simulink model "ControlsWithAutopilot_NoBus_PP_Discrete_Fcn_Atomic"  (Simulink 7.2)
settings: Solver=ode45  StartTime=0.0  StopTime=10.0  RelTol=1e-3
undefined symbols (not defined in the file): ap, bias, DiscIntNeverNeededParam
libraries: simulink x3, discretizing x1
(part 2 of 2)

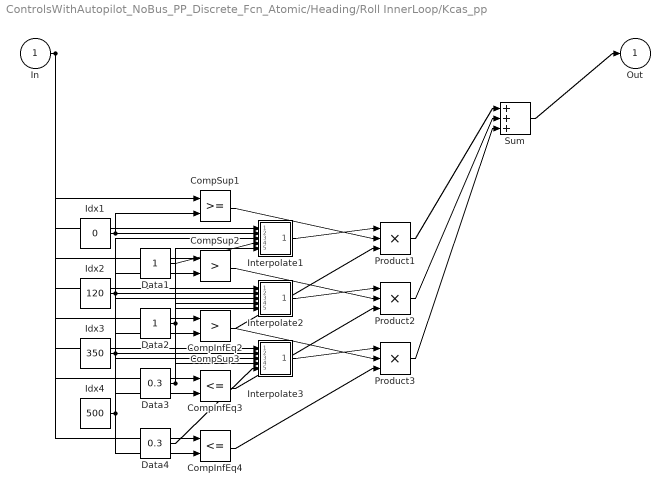
== system ControlsWithAutopilot_NoBus_PP_Discrete_Fcn_Atomic/Heading/Roll InnerLoop/Kcas_pp ==
  In : Inport
  CompInfEq2 : RelationalOperator  Operator=<=  InputSameDT=on
  CompInfEq3 : RelationalOperator  Operator=<=  InputSameDT=on
  CompInfEq4 : RelationalOperator  Operator=<=  InputSameDT=on
  CompSup1 : RelationalOperator  InputSameDT=on
  CompSup2 : RelationalOperator  Operator=>  InputSameDT=on
  CompSup3 : RelationalOperator  Operator=>  InputSameDT=on
  Data1 : Constant
  Data2 : Constant
  Data3 : Constant  Value=0.3
  Data4 : Constant  Value=0.3
  Idx1 : Constant  Value=0
  Idx2 : Constant  Value=120
  Idx3 : Constant  Value=350
  Idx4 : Constant  Value=500
  Interpolate1 : Subsystem
  Interpolate2 : Subsystem
  Interpolate3 : Subsystem
  Product1 : Product  Inputs=***  SaturateOnIntegerOverflow=on  RndMeth=Zero  OutDataTypeStr=Inherit: Same as first input
  Product2 : Product  Inputs=***  SaturateOnIntegerOverflow=on  RndMeth=Zero  OutDataTypeStr=Inherit: Same as first input
  Product3 : Product  Inputs=***  SaturateOnIntegerOverflow=on  RndMeth=Zero  OutDataTypeStr=Inherit: Same as first input
  Sum : Sum  Inputs=+++  SaturateOnIntegerOverflow=on  InputSameDT=on  OutDataTypeStr=Inherit: Same as first input
  Out : Outport
  wires:
  In/1 -> Interpolate1/1(InportIn), CompSup1/1, Interpolate2/1(InportIn), CompSup2/1, CompInfEq2/1, Interpolate3/1(InportIn), CompSup3/1, CompInfEq3/1, CompInfEq4/1
  Idx1/1 -> Interpolate1/2(InportIdx1), CompSup1/2
  Data1/1 -> Interpolate1/4(InportData1)
  Interpolate1/1(Out) -> Product1/1
  CompSup1/1 -> Product1/2
  CompInfEq2/1 -> Product1/3
  Product1/1 -> Sum/1
  Idx2/1 -> Interpolate2/2(InportIdx1), CompSup2/2, Interpolate1/3(InportIdx2), CompInfEq2/2
  Data2/1 -> Interpolate2/4(InportData1), Interpolate1/5(InportData2)
  Interpolate2/1(Out) -> Product2/1
  CompSup2/1 -> Product2/2
  CompInfEq3/1 -> Product2/3
  Product2/1 -> Sum/2
  Idx3/1 -> Interpolate3/2(InportIdx1), CompSup3/2, Interpolate2/3(InportIdx2), CompInfEq3/2
  Data3/1 -> Interpolate3/4(InportData1), Interpolate2/5(InportData2)
  Interpolate3/1(Out) -> Product3/1
  CompSup3/1 -> Product3/2
  CompInfEq4/1 -> Product3/3
  Product3/1 -> Sum/3
  Idx4/1 -> Interpolate3/3(InportIdx2), CompInfEq4/2
  Data4/1 -> Interpolate3/5(InportData2)
  Sum/1 -> Out/1

== system ControlsWithAutopilot_NoBus_PP_Discrete_Fcn_Atomic/Longitudinal/Altitude Control/Variable  Rate Limit ==
  ratelim : Inport  RequirementInfo={} %GIDa_1ef85aab_f902_404e_a68b_00e57673dd3f
  input : Inport  RequirementInfo={} %GIDa_7ac59940_1fcc_4039_a5aa_a007950c590e  Port=2
  ICtrig : Inport  RequirementInfo={} %GIDa_9850dee7_08ca_49d5_88fb_399ee4ba203e  Port=3
  IC : Inport  RequirementInfo={} %GIDa_d80fe626_91fd_4f82_ad17_86aca6b3aee5  Port=4
  Gain : Gain  RequirementInfo={} %GIDa_55467e41_3bd6_44bf_9a44_6f78661bf8f0  Gain=20  SaturateOnIntegerOverflow=on  OutDataTypeStr=Inherit: Same as input  ParamDataTypeStr=Inherit: Same as input
  Gain1 : Gain  RequirementInfo={} %GIDa_0b7dd2e9_dfcf_42d3_8fb1_8c254e005ceb  Gain=-1  SaturateOnIntegerOverflow=on  OutDataTypeStr=Inherit: Same as input  ParamDataTypeStr=Inherit: Same as input
  Integrator : DiscreteIntegrator  ExternalReset=level  InitialConditionSource=external  SampleTime=1.0  ICPrevOutput=DiscIntNeverNeededParam  ICPrevScaledInput=DiscIntNeverNeededParam  mask(DiscretizedDiscreteIntegrator){}
      mask init:
      | %zoh
  Sum2 : Sum  RequirementInfo={} %GIDa_de9ff84b_54f5_48bc_9ef3_874415208380  Inputs=|+-  SaturateOnIntegerOverflow=on
  Variable Limit Saturation : Subsystem  RequirementInfo={} %GIDa_42540829_63e9_4d83_adf5_d7c684208c2d
  output : Outport  RequirementInfo={} %GIDa_74eb2916_410f_4b2d_afdf_0d476e7e03b7
  wires:
  Sum2/1 -> Gain/1
  Gain/1 -> Variable Limit Saturation/2(SigIn)
  ratelim/1 -> Gain1/1, Variable Limit Saturation/1(up_lim)
  Gain1/1 -> Variable Limit Saturation/3(Lo_lim)
  Variable Limit Saturation/1(Out1) -> Integrator/1
  Integrator/1 -> Sum2/2, output/1
  input/1 -> Sum2/1
  ICtrig/1 -> Integrator/2
  IC/1 -> Integrator/3

== system ControlsWithAutopilot_NoBus_PP_Discrete_Fcn_Atomic/Longitudinal/Altitude Control/Variable Limit Saturation ==
  up_lim : Inport  RequirementInfo={} %GIDa_a8c5a358_1294_4ae6_a63f_3940fe218386
  SigIn : Inport  RequirementInfo={} %GIDa_062a0af8_40f0_4204_856b_8e0aded8de05  Port=2
  Lo_lim : Inport  RequirementInfo={} %GIDa_6793747b_c094_4bd9_a5cb_839f8eb54e21  Port=3
  Enforce low lim : MinMax  RequirementInfo={} %GIDa_e93f4b97_2f8b_4f52_84c9_3cb68ddf7e16  Function=max  Inputs=2
  Enforce up lim : MinMax  RequirementInfo={} %GIDa_c018e6ad_c664_4361_a96c_d990e2efb7d8  Inputs=2
  Out1 : Outport  RequirementInfo={} %GIDa_0d7a9d35_dde5_41a4_a708_f2de214bfa54
  wires:
  Lo_lim/1 -> Enforce low lim/1
  SigIn/1 -> Enforce low lim/2
  Enforce low lim/1 -> Enforce up lim/1
  up_lim/1 -> Enforce up lim/2
  Enforce up lim/1 -> Out1/1

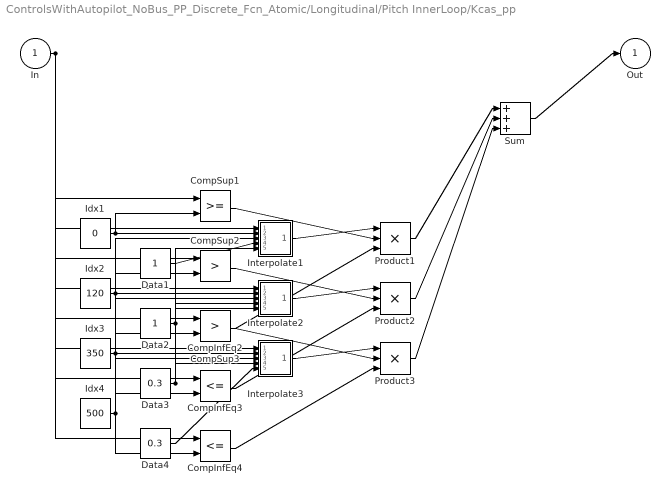
== system ControlsWithAutopilot_NoBus_PP_Discrete_Fcn_Atomic/Longitudinal/Pitch InnerLoop/Kcas_pp ==
  In : Inport
  CompInfEq2 : RelationalOperator  Operator=<=  InputSameDT=on
  CompInfEq3 : RelationalOperator  Operator=<=  InputSameDT=on
  CompInfEq4 : RelationalOperator  Operator=<=  InputSameDT=on
  CompSup1 : RelationalOperator  InputSameDT=on
  CompSup2 : RelationalOperator  Operator=>  InputSameDT=on
  CompSup3 : RelationalOperator  Operator=>  InputSameDT=on
  Data1 : Constant
  Data2 : Constant
  Data3 : Constant  Value=0.3
  Data4 : Constant  Value=0.3
  Idx1 : Constant  Value=0
  Idx2 : Constant  Value=120
  Idx3 : Constant  Value=350
  Idx4 : Constant  Value=500
  Interpolate1 : Subsystem
  Interpolate2 : Subsystem
  Interpolate3 : Subsystem
  Product1 : Product  Inputs=***  SaturateOnIntegerOverflow=on  RndMeth=Zero  OutDataTypeStr=Inherit: Same as first input
  Product2 : Product  Inputs=***  SaturateOnIntegerOverflow=on  RndMeth=Zero  OutDataTypeStr=Inherit: Same as first input
  Product3 : Product  Inputs=***  SaturateOnIntegerOverflow=on  RndMeth=Zero  OutDataTypeStr=Inherit: Same as first input
  Sum : Sum  Inputs=+++  SaturateOnIntegerOverflow=on  InputSameDT=on  OutDataTypeStr=Inherit: Same as first input
  Out : Outport
  wires:
  In/1 -> Interpolate1/1(InportIn), CompSup1/1, Interpolate2/1(InportIn), CompSup2/1, CompInfEq2/1, Interpolate3/1(InportIn), CompSup3/1, CompInfEq3/1, CompInfEq4/1
  Idx1/1 -> Interpolate1/2(InportIdx1), CompSup1/2
  Data1/1 -> Interpolate1/4(InportData1)
  Interpolate1/1(Out) -> Product1/1
  CompSup1/1 -> Product1/2
  CompInfEq2/1 -> Product1/3
  Product1/1 -> Sum/1
  Idx2/1 -> Interpolate2/2(InportIdx1), CompSup2/2, Interpolate1/3(InportIdx2), CompInfEq2/2
  Data2/1 -> Interpolate2/4(InportData1), Interpolate1/5(InportData2)
  Interpolate2/1(Out) -> Product2/1
  CompSup2/1 -> Product2/2
  CompInfEq3/1 -> Product2/3
  Product2/1 -> Sum/2
  Idx3/1 -> Interpolate3/2(InportIdx1), CompSup3/2, Interpolate2/3(InportIdx2), CompInfEq3/2
  Data3/1 -> Interpolate3/4(InportData1), Interpolate2/5(InportData2)
  Interpolate3/1(Out) -> Product3/1
  CompSup3/1 -> Product3/2
  CompInfEq4/1 -> Product3/3
  Product3/1 -> Sum/3
  Idx4/1 -> Interpolate3/3(InportIdx2), CompInfEq4/2
  Data4/1 -> Interpolate3/5(InportData2)
  Sum/1 -> Out/1

== system ControlsWithAutopilot_NoBus_PP_Discrete_Fcn_Atomic/Longitudinal/Pitch InnerLoop/Transfer Fcn_pp ==
  Inport1 : Inport
  D1 : UnitDelay  SampleTime=-1
  GainAC1_1 : Gain  Gain=-0.0625  SaturateOnIntegerOverflow=on  OutDataTypeStr=Inherit: Same as input  ParamDataTypeStr=Inherit: Same as input
  GainAC2_1 : Gain  Gain=-0.0625  SaturateOnIntegerOverflow=on  OutDataTypeStr=Inherit: Same as input  ParamDataTypeStr=Inherit: Same as input
  GainBD1_1 : Gain  SaturateOnIntegerOverflow=on  OutDataTypeStr=Inherit: Same as input  ParamDataTypeStr=Inherit: Same as input
  GainBD2_1 : Gain  SaturateOnIntegerOverflow=on  OutDataTypeStr=Inherit: Same as input  ParamDataTypeStr=Inherit: Same as input
  Sum1 : Sum  SaturateOnIntegerOverflow=on  InputSameDT=on  OutDataTypeStr=Inherit: Same as first input
  Sum2 : Sum  SaturateOnIntegerOverflow=on  InputSameDT=on  OutDataTypeStr=Inherit: Same as first input
  Outport1 : Outport
  wires:
  D1/1 -> GainAC1_1/1, GainAC2_1/1
  GainAC1_1/1 -> Sum1/1
  GainAC2_1/1 -> Sum2/1
  Inport1/1 -> GainBD1_1/1, GainBD2_1/1
  GainBD1_1/1 -> Sum1/2
  GainBD2_1/1 -> Sum2/2
  Sum1/1 -> D1/1
  Sum2/1 -> Outport1/1

== system ControlsWithAutopilot_NoBus_PP_Discrete_Fcn_Atomic/Yaw Damper/Kcas_pp/Interpolate1 ==
  InportIn : Inport
  InportIdx1 : Inport  Port=2
  InportIdx2 : Inport  Port=3
  InportData1 : Inport  Port=4
  InportData2 : Inport  Port=5
  Interpolate : Product  Inputs=*/*  SaturateOnIntegerOverflow=on  RndMeth=Zero  InputSameDT=on  OutDataTypeStr=Inherit: Same as first input
  Sum1 : Sum  Inputs=+-  SaturateOnIntegerOverflow=on  InputSameDT=on  OutDataTypeStr=Inherit: Same as first input
  Sum2 : Sum  Inputs=-+  SaturateOnIntegerOverflow=on  InputSameDT=on  OutDataTypeStr=Inherit: Same as first input
  Sum3 : Sum  Inputs=-+  SaturateOnIntegerOverflow=on  InputSameDT=on  OutDataTypeStr=Inherit: Same as first input
  Sum4 : Sum  SaturateOnIntegerOverflow=on  InputSameDT=on  OutDataTypeStr=Inherit: Same as first input
  Out : Outport
  wires:
  InportIn/1 -> Sum1/1
  InportIdx1/1 -> Sum1/2, Sum2/1
  InportIdx2/1 -> Sum2/2
  InportData1/1 -> Sum3/1, Sum4/2
  InportData2/1 -> Sum3/2
  Sum1/1 -> Interpolate/1
  Sum2/1 -> Interpolate/2
  Sum3/1 -> Interpolate/3
  Interpolate/1 -> Sum4/1
  Sum4/1 -> Out/1

== system ControlsWithAutopilot_NoBus_PP_Discrete_Fcn_Atomic/Yaw Damper/Kcas_pp/Interpolate2 ==
  InportIn : Inport
  InportIdx1 : Inport  Port=2
  InportIdx2 : Inport  Port=3
  InportData1 : Inport  Port=4
  InportData2 : Inport  Port=5
  Interpolate : Product  Inputs=*/*  SaturateOnIntegerOverflow=on  RndMeth=Zero  InputSameDT=on  OutDataTypeStr=Inherit: Same as first input
  Sum1 : Sum  Inputs=+-  SaturateOnIntegerOverflow=on  InputSameDT=on  OutDataTypeStr=Inherit: Same as first input
  Sum2 : Sum  Inputs=-+  SaturateOnIntegerOverflow=on  InputSameDT=on  OutDataTypeStr=Inherit: Same as first input
  Sum3 : Sum  Inputs=-+  SaturateOnIntegerOverflow=on  InputSameDT=on  OutDataTypeStr=Inherit: Same as first input
  Sum4 : Sum  SaturateOnIntegerOverflow=on  InputSameDT=on  OutDataTypeStr=Inherit: Same as first input
  Out : Outport
  wires:
  InportIn/1 -> Sum1/1
  InportIdx1/1 -> Sum1/2, Sum2/1
  InportIdx2/1 -> Sum2/2
  InportData1/1 -> Sum3/1, Sum4/2
  InportData2/1 -> Sum3/2
  Sum1/1 -> Interpolate/1
  Sum2/1 -> Interpolate/2
  Sum3/1 -> Interpolate/3
  Interpolate/1 -> Sum4/1
  Sum4/1 -> Out/1

== system ControlsWithAutopilot_NoBus_PP_Discrete_Fcn_Atomic/Yaw Damper/Kcas_pp/Interpolate3 ==
  InportIn : Inport
  InportIdx1 : Inport  Port=2
  InportIdx2 : Inport  Port=3
  InportData1 : Inport  Port=4
  InportData2 : Inport  Port=5
  Interpolate : Product  Inputs=*/*  SaturateOnIntegerOverflow=on  RndMeth=Zero  InputSameDT=on  OutDataTypeStr=Inherit: Same as first input
  Sum1 : Sum  Inputs=+-  SaturateOnIntegerOverflow=on  InputSameDT=on  OutDataTypeStr=Inherit: Same as first input
  Sum2 : Sum  Inputs=-+  SaturateOnIntegerOverflow=on  InputSameDT=on  OutDataTypeStr=Inherit: Same as first input
  Sum3 : Sum  Inputs=-+  SaturateOnIntegerOverflow=on  InputSameDT=on  OutDataTypeStr=Inherit: Same as first input
  Sum4 : Sum  SaturateOnIntegerOverflow=on  InputSameDT=on  OutDataTypeStr=Inherit: Same as first input
  Out : Outport
  wires:
  InportIn/1 -> Sum1/1
  InportIdx1/1 -> Sum1/2, Sum2/1
  InportIdx2/1 -> Sum2/2
  InportData1/1 -> Sum3/1, Sum4/2
  InportData2/1 -> Sum3/2
  Sum1/1 -> Interpolate/1
  Sum2/1 -> Interpolate/2
  Sum3/1 -> Interpolate/3
  Interpolate/1 -> Sum4/1
  Sum4/1 -> Out/1

== system ControlsWithAutopilot_NoBus_PP_Discrete_Fcn_Atomic/Heading/Heading Control/HdgCmdProcessor/ANGL ==
  in : Inport  RequirementInfo={} %GIDa_91f853c7_c908_401d_adfc_518d7751528f
  Abs : Abs  OutDataType=sfix(16)  OutScaling=2^0
  Constant : Constant  Value=360  OutDataType=sfix(16)  OutScaling=2^0
  Constant1 : Constant  RequirementInfo={} %GIDa_7c5c3c02_b72b_4cab_88d9_ce8964dea6e5  Value=180
  Product : Product  OutDataType=sfix(16)  OutScaling=2^0  RndMeth=Zero
  Relational Operator : RelationalOperator  RequirementInfo={} %GIDa_7fca63f4_30c3_4611_a13c_f242258541ac  Operator=>
  Relational Operator1 : RelationalOperator  Operator=<  LogicOutDataTypeMode=boolean  OutDataTypeStr=boolean
  Sum6 : Sum  RequirementInfo={} %GIDa_8f691f86_6b2c_4343_a08d_01121fff99a8  Inputs=|-+  SaturateOnIntegerOverflow=on
  Switch1 : Switch  RequirementInfo={} %GIDa_9f6a3e17_ac1f_4a7c_b770_43e31d539b0d  Threshold=0.1  SaturateOnIntegerOverflow=on
  zero : Constant  Value=0  OutDataType=sfix(16)  OutScaling=2^0
  180 : Outport  RequirementInfo={} %GIDa_da671ccf_1469_4f90_9911_e50416dafc2f
  wires:
  Abs/1 -> Relational Operator/1
  in/1 -> Abs/1, Switch1/3, Sum6/2, Relational Operator1/2
  Switch1/1 -> 180/1
  Product/1 -> Sum6/1
  Sum6/1 -> Switch1/1
  Relational Operator/1 -> Switch1/2
  Constant1/1 -> Relational Operator/2
  zero/1 -> Relational Operator1/1
  Constant/1 -> Product/1
  Relational Operator1/1 -> Product/2

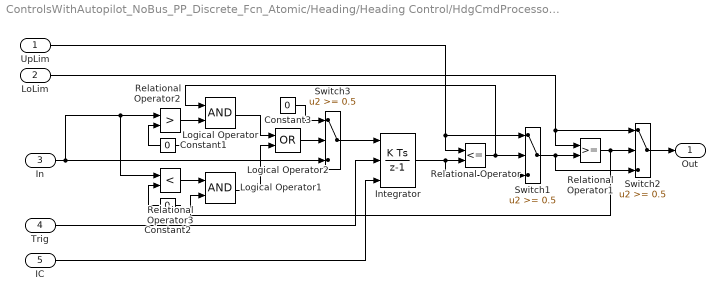
== system ControlsWithAutopilot_NoBus_PP_Discrete_Fcn_Atomic/Heading/Heading Control/HdgCmdProcessor/VarLimIntegIC ==
  UpLim : Inport  RequirementInfo={} %GIDa_b6974814_32b4_446c_a7b5_2b64616822d2
  LoLim : Inport  RequirementInfo={} %GIDa_b4069f0f_04d2_435d_9d74_47f31e226abc  Port=2
  In : Inport  RequirementInfo={} %GIDa_ffe63698_9663_4b08_a6c4_0cfcc14ab018  Port=3
  Trig : Inport  RequirementInfo={} %GIDa_6297cb9d_5b31_4d8e_a321_41fbf142c5b4  Port=4
  IC : Inport  RequirementInfo={} %GIDa_59f2d505_3cc2_4942_9dd8_a5a4ff923eba  Port=5
  Constant1 : Constant  RequirementInfo={} %GIDa_5f63bf18_9b52_4c75_b33f_d083ba316d1e  Value=0
  Constant2 : Constant  RequirementInfo={} %GIDa_3ef1a0c3_325a_4a1e_87f1_8a7ceb7f2ed7  Value=0
  Constant3 : Constant  RequirementInfo={} %GIDa_3c010cc6_e66d_42da_9a5a_231ebe5e9c3f  Value=0
  Integrator : DiscreteIntegrator  ExternalReset=level  InitialConditionSource=external  SampleTime=1.0  ICPrevOutput=DiscIntNeverNeededParam  ICPrevScaledInput=DiscIntNeverNeededParam  mask(DiscretizedDiscreteIntegrator){}
      mask init:
      | %zoh
  Logical Operator : Logic  RequirementInfo={} %GIDa_a60b4d2f_6552_4cb5_b522_727de66498b0  AllPortsSameDT=off
  Logical Operator1 : Logic  RequirementInfo={} %GIDa_8f81d6cf_a2aa_4e00_869d_ceffbd7871c1  AllPortsSameDT=off
  Logical Operator2 : Logic  RequirementInfo={} %GIDa_6338745d_e0be_46bf_a46f_644f808dad4e  Operator=OR  AllPortsSameDT=off
  Relational Operator : RelationalOperator  RequirementInfo={} %GIDa_8e878cd0_b3b2_4162_9fe2_c686049f0806  Operator=<=
  Relational Operator1 : RelationalOperator  RequirementInfo={} %GIDa_b45a0ded_1a8c_4a6d_a67f_e5d263373459
  Relational Operator2 : RelationalOperator  RequirementInfo={} %GIDa_a0755ed8_a69f_4262_8ce5_c41fc56502ff  Operator=>
  Relational Operator3 : RelationalOperator  RequirementInfo={} %GIDa_8264758e_f6c1_4924_85b8_a6eda5126d21  Operator=<
  Switch1 : Switch  RequirementInfo={} %GIDa_4c3fce01_41f9_40b1_a6a3_6d04c9eccd5a  Threshold=0.5  SaturateOnIntegerOverflow=on  InputSameDT=on
  Switch2 : Switch  RequirementInfo={} %GIDa_b2e7bf7c_7029_45e6_9cda_915a12f41445  Threshold=0.5  SaturateOnIntegerOverflow=on  InputSameDT=on
  Switch3 : Switch  RequirementInfo={} %GIDa_bec6d583_cd7d_4a0e_9481_7e8d505e2b66  Threshold=0.5  SaturateOnIntegerOverflow=on  InputSameDT=on
  Out : Outport  RequirementInfo={} %GIDa_6b54eae4_0c2d_43e8_87f0_b15564168c0d
  wires:
  Relational Operator1/1 -> Logical Operator1/2, Switch2/2
  Switch1/1 -> Switch2/3, Relational Operator1/2
  LoLim/1 -> Relational Operator1/1, Switch2/1
  IC/1 -> Integrator/3
  Trig/1 -> Integrator/2
  Constant2/1 -> Relational Operator3/2
  Relational Operator3/1 -> Logical Operator1/1
  Logical Operator1/1 -> Logical Operator2/2
  Logical Operator/1 -> Logical Operator2/1
  Logical Operator2/1 -> Switch3/2
  Relational Operator2/1 -> Logical Operator/2
  Constant1/1 -> Relational Operator2/2
  In/1 -> Switch3/3, Relational Operator3/1, Relational Operator2/1
  Constant3/1 -> Switch3/1
  Switch3/1 -> Integrator/1
  Relational Operator/1 -> Logical Operator/1, Switch1/2
  Switch2/1 -> Out/1
  UpLim/1 -> Switch1/1, Relational Operator/1
  Integrator/1 -> Relational Operator/2, Switch1/3

== system ControlsWithAutopilot_NoBus_PP_Discrete_Fcn_Atomic/Heading/Roll InnerLoop/Kcas_pp/Interpolate1 ==
  InportIn : Inport
  InportIdx1 : Inport  Port=2
  InportIdx2 : Inport  Port=3
  InportData1 : Inport  Port=4
  InportData2 : Inport  Port=5
  Interpolate : Product  Inputs=*/*  SaturateOnIntegerOverflow=on  RndMeth=Zero  InputSameDT=on  OutDataTypeStr=Inherit: Same as first input
  Sum1 : Sum  Inputs=+-  SaturateOnIntegerOverflow=on  InputSameDT=on  OutDataTypeStr=Inherit: Same as first input
  Sum2 : Sum  Inputs=-+  SaturateOnIntegerOverflow=on  InputSameDT=on  OutDataTypeStr=Inherit: Same as first input
  Sum3 : Sum  Inputs=-+  SaturateOnIntegerOverflow=on  InputSameDT=on  OutDataTypeStr=Inherit: Same as first input
  Sum4 : Sum  SaturateOnIntegerOverflow=on  InputSameDT=on  OutDataTypeStr=Inherit: Same as first input
  Out : Outport
  wires:
  InportIn/1 -> Sum1/1
  InportIdx1/1 -> Sum1/2, Sum2/1
  InportIdx2/1 -> Sum2/2
  InportData1/1 -> Sum3/1, Sum4/2
  InportData2/1 -> Sum3/2
  Sum1/1 -> Interpolate/1
  Sum2/1 -> Interpolate/2
  Sum3/1 -> Interpolate/3
  Interpolate/1 -> Sum4/1
  Sum4/1 -> Out/1

== system ControlsWithAutopilot_NoBus_PP_Discrete_Fcn_Atomic/Heading/Roll InnerLoop/Kcas_pp/Interpolate2 ==
  InportIn : Inport
  InportIdx1 : Inport  Port=2
  InportIdx2 : Inport  Port=3
  InportData1 : Inport  Port=4
  InportData2 : Inport  Port=5
  Interpolate : Product  Inputs=*/*  SaturateOnIntegerOverflow=on  RndMeth=Zero  InputSameDT=on  OutDataTypeStr=Inherit: Same as first input
  Sum1 : Sum  Inputs=+-  SaturateOnIntegerOverflow=on  InputSameDT=on  OutDataTypeStr=Inherit: Same as first input
  Sum2 : Sum  Inputs=-+  SaturateOnIntegerOverflow=on  InputSameDT=on  OutDataTypeStr=Inherit: Same as first input
  Sum3 : Sum  Inputs=-+  SaturateOnIntegerOverflow=on  InputSameDT=on  OutDataTypeStr=Inherit: Same as first input
  Sum4 : Sum  SaturateOnIntegerOverflow=on  InputSameDT=on  OutDataTypeStr=Inherit: Same as first input
  Out : Outport
  wires:
  InportIn/1 -> Sum1/1
  InportIdx1/1 -> Sum1/2, Sum2/1
  InportIdx2/1 -> Sum2/2
  InportData1/1 -> Sum3/1, Sum4/2
  InportData2/1 -> Sum3/2
  Sum1/1 -> Interpolate/1
  Sum2/1 -> Interpolate/2
  Sum3/1 -> Interpolate/3
  Interpolate/1 -> Sum4/1
  Sum4/1 -> Out/1

== system ControlsWithAutopilot_NoBus_PP_Discrete_Fcn_Atomic/Heading/Roll InnerLoop/Kcas_pp/Interpolate3 ==
  InportIn : Inport
  InportIdx1 : Inport  Port=2
  InportIdx2 : Inport  Port=3
  InportData1 : Inport  Port=4
  InportData2 : Inport  Port=5
  Interpolate : Product  Inputs=*/*  SaturateOnIntegerOverflow=on  RndMeth=Zero  InputSameDT=on  OutDataTypeStr=Inherit: Same as first input
  Sum1 : Sum  Inputs=+-  SaturateOnIntegerOverflow=on  InputSameDT=on  OutDataTypeStr=Inherit: Same as first input
  Sum2 : Sum  Inputs=-+  SaturateOnIntegerOverflow=on  InputSameDT=on  OutDataTypeStr=Inherit: Same as first input
  Sum3 : Sum  Inputs=-+  SaturateOnIntegerOverflow=on  InputSameDT=on  OutDataTypeStr=Inherit: Same as first input
  Sum4 : Sum  SaturateOnIntegerOverflow=on  InputSameDT=on  OutDataTypeStr=Inherit: Same as first input
  Out : Outport
  wires:
  InportIn/1 -> Sum1/1
  InportIdx1/1 -> Sum1/2, Sum2/1
  InportIdx2/1 -> Sum2/2
  InportData1/1 -> Sum3/1, Sum4/2
  InportData2/1 -> Sum3/2
  Sum1/1 -> Interpolate/1
  Sum2/1 -> Interpolate/2
  Sum3/1 -> Interpolate/3
  Interpolate/1 -> Sum4/1
  Sum4/1 -> Out/1

== system ControlsWithAutopilot_NoBus_PP_Discrete_Fcn_Atomic/Longitudinal/Altitude Control/Variable  Rate Limit/Variable Limit Saturation ==
  up_lim : Inport  RequirementInfo={} %GIDa_c3426702_ae57_4a6b_8e5b_d8e7ea7997b8
  SigIn : Inport  RequirementInfo={} %GIDa_57ffe4bd_514b_4f1d_925b_ea07d6710330  Port=2
  Lo_lim : Inport  RequirementInfo={} %GIDa_934c3ebb_c2a8_4cb2_b1d4_7a7b38287908  Port=3
  Enforce low lim : MinMax  RequirementInfo={} %GIDa_f320f771_b833_4e25_ab12_e91693dd9b04  Function=max  Inputs=2
  Enforce up lim : MinMax  RequirementInfo={} %GIDa_1cfdde9a_faa1_4e7e_9516_cacb3f0cb773  Inputs=2
  Out1 : Outport  RequirementInfo={} %GIDa_6b324e36_3b21_43eb_ae92_bdd39356922a
  wires:
  Enforce up lim/1 -> Out1/1
  up_lim/1 -> Enforce up lim/2
  Enforce low lim/1 -> Enforce up lim/1
  SigIn/1 -> Enforce low lim/2
  Lo_lim/1 -> Enforce low lim/1

== system ControlsWithAutopilot_NoBus_PP_Discrete_Fcn_Atomic/Longitudinal/Pitch InnerLoop/Kcas_pp/Interpolate1 ==
  InportIn : Inport
  InportIdx1 : Inport  Port=2
  InportIdx2 : Inport  Port=3
  InportData1 : Inport  Port=4
  InportData2 : Inport  Port=5
  Interpolate : Product  Inputs=*/*  SaturateOnIntegerOverflow=on  RndMeth=Zero  InputSameDT=on  OutDataTypeStr=Inherit: Same as first input
  Sum1 : Sum  Inputs=+-  SaturateOnIntegerOverflow=on  InputSameDT=on  OutDataTypeStr=Inherit: Same as first input
  Sum2 : Sum  Inputs=-+  SaturateOnIntegerOverflow=on  InputSameDT=on  OutDataTypeStr=Inherit: Same as first input
  Sum3 : Sum  Inputs=-+  SaturateOnIntegerOverflow=on  InputSameDT=on  OutDataTypeStr=Inherit: Same as first input
  Sum4 : Sum  SaturateOnIntegerOverflow=on  InputSameDT=on  OutDataTypeStr=Inherit: Same as first input
  Out : Outport
  wires:
  InportIn/1 -> Sum1/1
  InportIdx1/1 -> Sum1/2, Sum2/1
  InportIdx2/1 -> Sum2/2
  InportData1/1 -> Sum3/1, Sum4/2
  InportData2/1 -> Sum3/2
  Sum1/1 -> Interpolate/1
  Sum2/1 -> Interpolate/2
  Sum3/1 -> Interpolate/3
  Interpolate/1 -> Sum4/1
  Sum4/1 -> Out/1

== system ControlsWithAutopilot_NoBus_PP_Discrete_Fcn_Atomic/Longitudinal/Pitch InnerLoop/Kcas_pp/Interpolate2 ==
  InportIn : Inport
  InportIdx1 : Inport  Port=2
  InportIdx2 : Inport  Port=3
  InportData1 : Inport  Port=4
  InportData2 : Inport  Port=5
  Interpolate : Product  Inputs=*/*  SaturateOnIntegerOverflow=on  RndMeth=Zero  InputSameDT=on  OutDataTypeStr=Inherit: Same as first input
  Sum1 : Sum  Inputs=+-  SaturateOnIntegerOverflow=on  InputSameDT=on  OutDataTypeStr=Inherit: Same as first input
  Sum2 : Sum  Inputs=-+  SaturateOnIntegerOverflow=on  InputSameDT=on  OutDataTypeStr=Inherit: Same as first input
  Sum3 : Sum  Inputs=-+  SaturateOnIntegerOverflow=on  InputSameDT=on  OutDataTypeStr=Inherit: Same as first input
  Sum4 : Sum  SaturateOnIntegerOverflow=on  InputSameDT=on  OutDataTypeStr=Inherit: Same as first input
  Out : Outport
  wires:
  InportIn/1 -> Sum1/1
  InportIdx1/1 -> Sum1/2, Sum2/1
  InportIdx2/1 -> Sum2/2
  InportData1/1 -> Sum3/1, Sum4/2
  InportData2/1 -> Sum3/2
  Sum1/1 -> Interpolate/1
  Sum2/1 -> Interpolate/2
  Sum3/1 -> Interpolate/3
  Interpolate/1 -> Sum4/1
  Sum4/1 -> Out/1

== system ControlsWithAutopilot_NoBus_PP_Discrete_Fcn_Atomic/Longitudinal/Pitch InnerLoop/Kcas_pp/Interpolate3 ==
  InportIn : Inport
  InportIdx1 : Inport  Port=2
  InportIdx2 : Inport  Port=3
  InportData1 : Inport  Port=4
  InportData2 : Inport  Port=5
  Interpolate : Product  Inputs=*/*  SaturateOnIntegerOverflow=on  RndMeth=Zero  InputSameDT=on  OutDataTypeStr=Inherit: Same as first input
  Sum1 : Sum  Inputs=+-  SaturateOnIntegerOverflow=on  InputSameDT=on  OutDataTypeStr=Inherit: Same as first input
  Sum2 : Sum  Inputs=-+  SaturateOnIntegerOverflow=on  InputSameDT=on  OutDataTypeStr=Inherit: Same as first input
  Sum3 : Sum  Inputs=-+  SaturateOnIntegerOverflow=on  InputSameDT=on  OutDataTypeStr=Inherit: Same as first input
  Sum4 : Sum  SaturateOnIntegerOverflow=on  InputSameDT=on  OutDataTypeStr=Inherit: Same as first input
  Out : Outport
  wires:
  InportIn/1 -> Sum1/1
  InportIdx1/1 -> Sum1/2, Sum2/1
  InportIdx2/1 -> Sum2/2
  InportData1/1 -> Sum3/1, Sum4/2
  InportData2/1 -> Sum3/2
  Sum1/1 -> Interpolate/1
  Sum2/1 -> Interpolate/2
  Sum3/1 -> Interpolate/3
  Interpolate/1 -> Sum4/1
  Sum4/1 -> Out/1
